simulink model "fuzzy control"  (R2021b)
settings: Solver=FixedStepAuto  StartTime=0.0  StopTime=500  FixedStep=0.1  RelTol=1e-3
libraries: simulink_extras x4, fuzblock x1
settings Model: Creator=扎尔  LastModifiedBy=扎尔

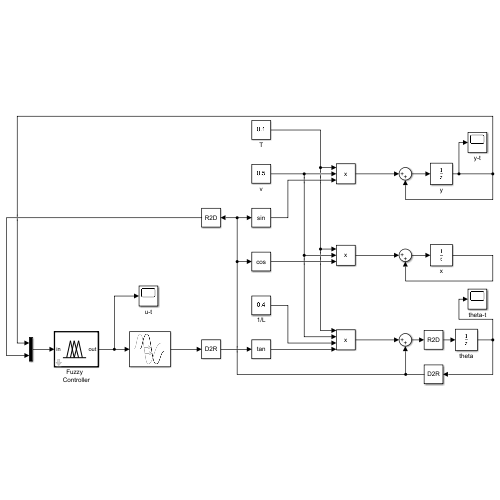
[thumbnail: Simulink's stored preview of the top-level diagram]
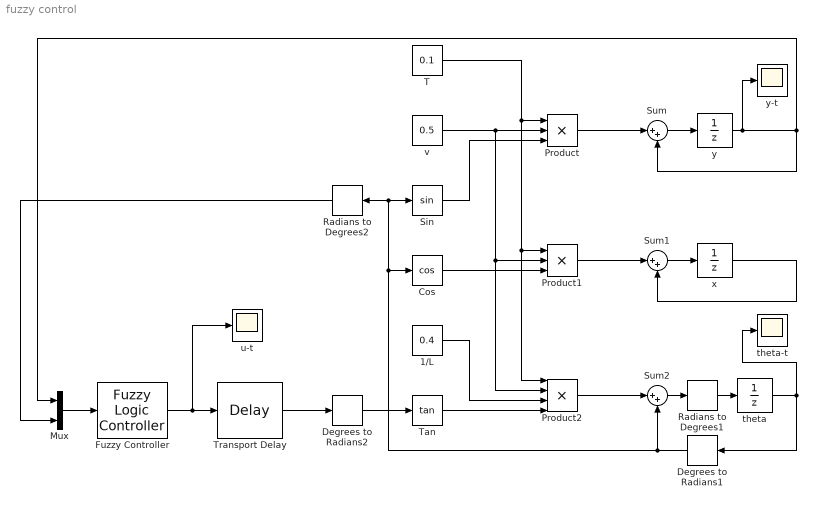
== system fuzzy control ==
  1/L : Constant  Value=0.4
  Cos : Trigonometry  Operator=cos
  Degrees to Radians1 : simulink_extras/Transformations/Degrees to Radians
  Degrees to Radians2 : simulink_extras/Transformations/Degrees to Radians
  Fuzzy Controller : fuzblock/Fuzzy Logic  Controller  FIS="\"fuzzy controller.fis\""  OutputSampleNumber=101  DataType=double  FuzzifiedInputs=off  RuleFiringStrengths=off  RuleOutputs=off  AggregatedOutputs=off  SimulateUsing=Interpreted execution  OutOfRangeInputValueMessage=warning  NoRuleFiredMessage=warning  EmptyOutputFuzzySetMessage=warning
  Mux : Mux  Inputs=2
  Product : Product  Inputs=3
  Product1 : Product  Inputs=3
  Product2 : Product  Inputs=4
  Radians to Degrees1 : simulink_extras/Transformations/Radians to Degrees
  Radians to Degrees2 : simulink_extras/Transformations/Radians to Degrees
  Sin : Trigonometry
  Sum : Sum  Inputs=|++
  Sum1 : Sum  Inputs=|++
  Sum2 : Sum  Inputs=|++
  T : Constant  Value=0.1
  Tan : Trigonometry  Operator=tan
  Transport Delay : TransportDelay  FixedBuffer=on
  theta : UnitDelay  SampleTime=-1  HasFrameUpgradeWarning=on
  theta-t : Scope
  u-t : Scope
  v : Constant  Value=0.5
  x : UnitDelay  InitialCondition=20  SampleTime=-1  HasFrameUpgradeWarning=on
  y : UnitDelay  InitialCondition=40  SampleTime=-1  HasFrameUpgradeWarning=on
  y-t : Scope
  wires:
  Mux/1 -> Fuzzy Controller/1
  Fuzzy Controller/1 -> u-t/1, Transport Delay/1
  v/1 -> Product1/2, Product2/2, Product/2
  T/1 -> Product2/1, Product1/1, Product/1
  Sin/1 -> Product/3
  Product/1 -> Sum/1
  Sum/1 -> y/1
  y/1 -> y-t/1, Sum/2, Mux/1
  Cos/1 -> Product1/3
  Product1/1 -> Sum1/1
  Sum1/1 -> x/1
  x/1 -> Sum1/2
  1/L/1 -> Product2/3
  Tan/1 -> Product2/4
  Product2/1 -> Sum2/1
  Transport Delay/1 -> Degrees to Radians2/1
  Sum2/1 -> Radians to Degrees1/1
  Radians to Degrees1/1 -> theta/1
  theta/1 -> theta-t/1, Degrees to Radians1/1
  Degrees to Radians2/1 -> Tan/1
  Radians to Degrees2/1 -> Mux/2
  Degrees to Radians1/1 -> Sum2/2, Cos/1, Sin/1, Radians to Degrees2/1
